simulink model "LQR_Simulink_Model"  (R2021a)
settings: Solver=VariableStepAuto  StartTime=0.0  StopTime=30  RelTol=1e-3
values from neighbouring files (symbols this model uses):
  f = 0.01    [modeling.m]
  g = 9.81    [modeling.m]
  I_pend = 0.00024    [modeling.m]
  K = K/v_to_force    [modeling.m]
  l = 0.04    [modeling.m]
  m_cart = 0.493    [modeling.m]
  m_pend = 0.312    [modeling.m]
libraries: simulink x1
settings Model: Creator=navoditchandra  LastModifiedBy=INEEDHEALING
settings DebuggingCC: UnderSpecifiedDimensionMsg=warning

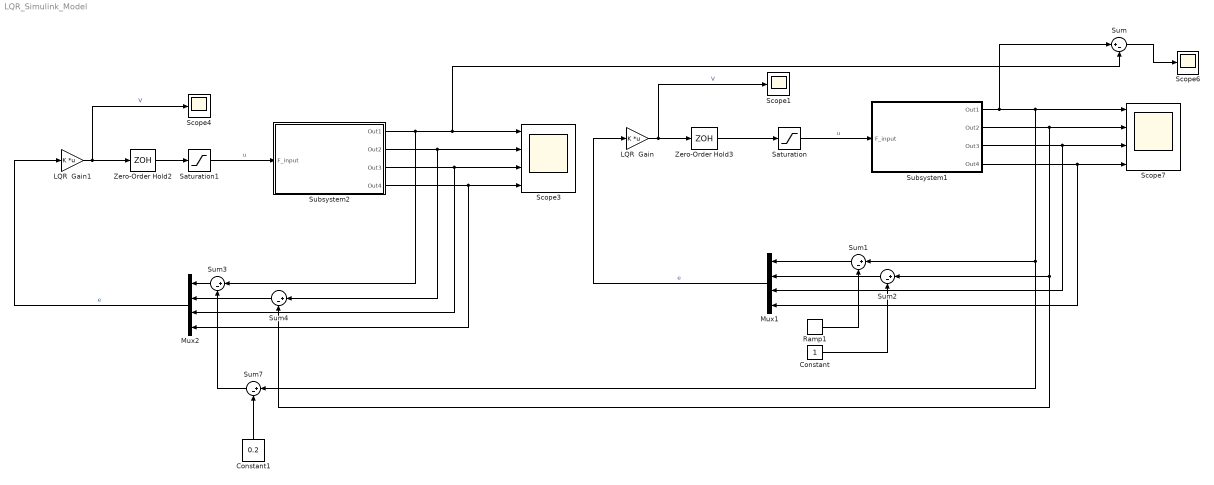
== system LQR_Simulink_Model ==
  Constant : Constant
  Constant1 : Constant  Value=0.2
  LQR  Gain : Gain  Gain=K  Multiplication=Matrix(K*u)
  LQR  Gain1 : Gain  Gain=K  Multiplication=Matrix(K*u)
  Mux1 : Mux
  Mux2 : Mux
  Ramp1 : simulink/Sources/Ramp  slope=1  start=0  InitialOutput=0
  Saturation : Saturate  UpperLimit=5  LowerLimit=-5
  Saturation1 : Saturate  UpperLimit=5  LowerLimit=-5
  Scope1 : Scope
  Scope3 : Scope  NumInputPorts=4
  Scope4 : Scope
  Scope6 : Scope
  Scope7 : Scope  NumInputPorts=4
  Subsystem1 : Subsystem
  Subsystem2 : Subsystem
  Sum{,1..4,7} (6 alike) : Sum  Inputs=|+-
  Zero-Order Hold2 : ZeroOrderHold  SampleTime=0.01
  Zero-Order Hold3 : ZeroOrderHold  SampleTime=0.01
  wires:
  Sum4/1 -> Mux2/2
  Sum3/1 -> Mux2/1
  Subsystem1/2(Out2) -> Scope7/2, Sum2/1, Sum4/2
  Mux1/1 -> LQR  Gain/1  "e"
  Subsystem1/4(Out4) -> Scope7/4, Mux1/4
  Saturation1/1 -> Subsystem2/1(F_input)  "u"
  Ramp1/1 -> Sum1/2
  Subsystem2/4(Out4) -> Mux2/4, Scope3/4
  Subsystem2/3(Out3) -> Mux2/3, Scope3/3
  Sum2/1 -> Mux1/2
  Mux2/1 -> LQR  Gain1/1  "e"
  Subsystem1/3(Out3) -> Scope7/3, Mux1/3
  Subsystem2/1(Out1) -> Scope3/1, Sum/2, Sum3/1
  Sum/1 -> Scope6/1
  Sum1/1 -> Mux1/1
  Subsystem2/2(Out2) -> Sum4/1, Scope3/2
  Subsystem1/1(Out1) -> Scope7/1, Sum7/1, Sum1/1, Sum/1
  Saturation/1 -> Subsystem1/1(F_input)  "u"
  Constant/1 -> Sum2/2
  Sum7/1 -> Sum3/2
  Constant1/1 -> Sum7/2
  LQR  Gain1/1 -> Scope4/1, Zero-Order Hold2/1  "V"
  Zero-Order Hold2/1 -> Saturation1/1
  LQR  Gain/1 -> Scope1/1, Zero-Order Hold3/1  "V"
  Zero-Order Hold3/1 -> Saturation/1

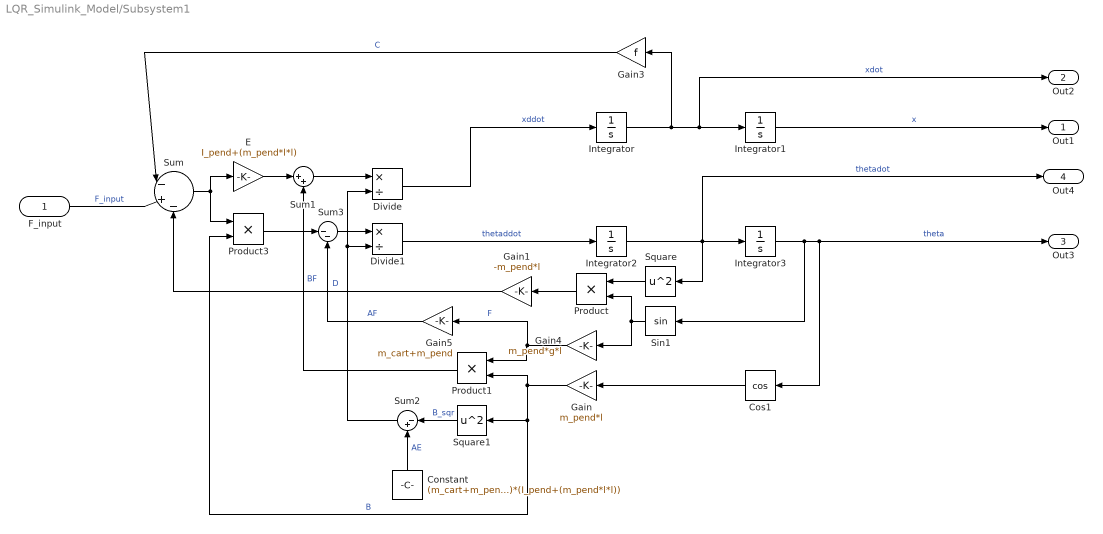
== system LQR_Simulink_Model/Subsystem1 ==
  F_input : Inport
  Constant : Constant  Value=(m_cart+m_pend)*(I_pend+(m_pend*l*l))
  Cos1 : Trigonometry  Operator=cos
  Divide : Product  Inputs=*/
  Divide1 : Product  Inputs=*/
  E : Gain  Gain=I_pend+(m_pend*l*l)
  Gain : Gain  Gain=m_pend*l
  Gain1 : Gain  Gain=-m_pend*l
  Gain3 : Gain  Gain=f
  Gain4 : Gain  Gain=m_pend*g*l
  Gain5 : Gain  Gain=m_cart+m_pend
  Integrator{,1..3} (4 alike) : Integrator
  Product : Product
  Product1 : Product
  Product3 : Product
  Sin1 : Trigonometry
  Square : Math  Operator=square  SaturateOnIntegerOverflow=on
  Square1 : Math  Operator=square  SaturateOnIntegerOverflow=on
  Sum : Sum  Inputs=|-+-
  Sum1 : Sum  Inputs=|++
  Sum2 : Sum  Inputs=|-+
  Sum3 : Sum  Inputs=|--
  Out1 : Outport
  Out2 : Outport  Port=2
  Out3 : Outport  Port=3
  Out4 : Outport  Port=4
  wires:
  Integrator2/1 -> Out4/1, Integrator3/1, Square/1  "thetadot"
  Integrator/1 -> Gain3/1, Integrator1/1, Out2/1  "xdot"
  Divide/1 -> Integrator/1  "xddot"
  Divide1/1 -> Integrator2/1  "thetaddot"
  Integrator1/1 -> Out1/1  "x"
  Gain/1 -> Product1/2, Product3/2, Square1/1  "B"
  Cos1/1 -> Gain/1
  Integrator3/1 -> Out3/1, Cos1/1, Sin1/1  "theta"
  Gain3/1 -> Sum/1  "C"
  Sin1/1 -> Gain4/1, Product/2
  Square/1 -> Product/1
  Product/1 -> Gain1/1
  Gain1/1 -> Sum/3  "D"
  Gain4/1 -> Gain5/1, Product1/1  "F"
  F_input/1 -> Sum/2  "F_input"
  Sum/1 -> Product3/1, E/1
  E/1 -> Sum1/1
  Product1/1 -> Sum1/2  "BF"
  Sum1/1 -> Divide/1
  Square1/1 -> Sum2/1  "B_sqr"
  Constant/1 -> Sum2/2  "AE"
  Sum2/1 -> Divide/2, Divide1/2
  Product3/1 -> Sum3/1
  Gain5/1 -> Sum3/2  "AF"
  Sum3/1 -> Divide1/1

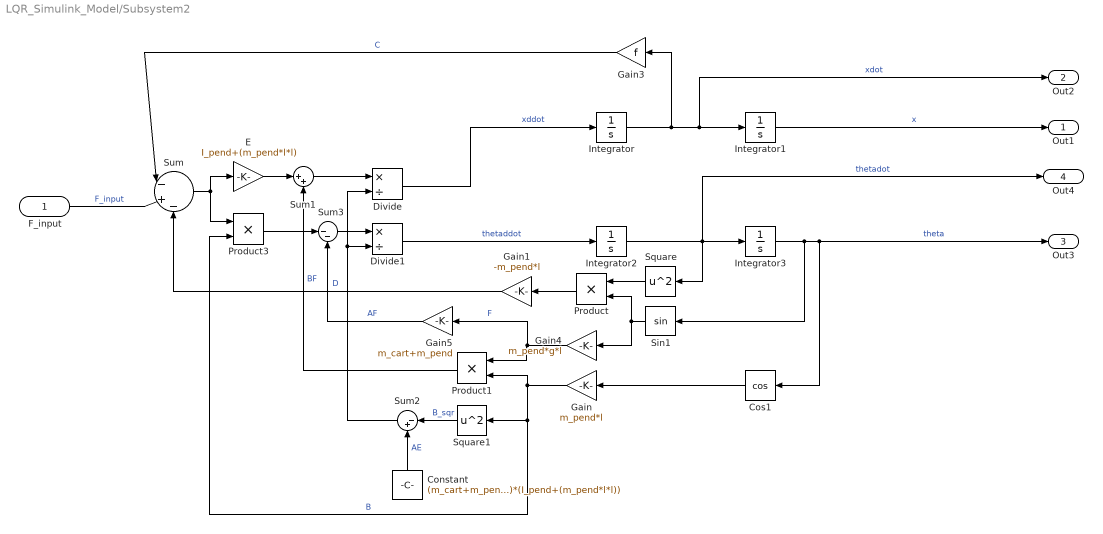
== system LQR_Simulink_Model/Subsystem2 ==
  F_input : Inport
  Constant : Constant  Value=(m_cart+m_pend)*(I_pend+(m_pend*l*l))
  Cos1 : Trigonometry  Operator=cos
  Divide : Product  Inputs=*/
  Divide1 : Product  Inputs=*/
  E : Gain  Gain=I_pend+(m_pend*l*l)
  Gain : Gain  Gain=m_pend*l
  Gain1 : Gain  Gain=-m_pend*l
  Gain3 : Gain  Gain=f
  Gain4 : Gain  Gain=m_pend*g*l
  Gain5 : Gain  Gain=m_cart+m_pend
  Integrator : Integrator
  Integrator1 : Integrator  InitialCondition=-0.2
  Integrator2 : Integrator
  Integrator3 : Integrator
  Product : Product
  Product1 : Product
  Product3 : Product
  Sin1 : Trigonometry
  Square : Math  Operator=square  SaturateOnIntegerOverflow=on
  Square1 : Math  Operator=square  SaturateOnIntegerOverflow=on
  Sum : Sum  Inputs=|-+-
  Sum1 : Sum  Inputs=|++
  Sum2 : Sum  Inputs=|-+
  Sum3 : Sum  Inputs=|--
  Out1 : Outport
  Out2 : Outport  Port=2
  Out3 : Outport  Port=3
  Out4 : Outport  Port=4
  wires:
  Integrator2/1 -> Out4/1, Integrator3/1, Square/1  "thetadot"
  Integrator/1 -> Gain3/1, Integrator1/1, Out2/1  "xdot"
  Divide/1 -> Integrator/1  "xddot"
  Divide1/1 -> Integrator2/1  "thetaddot"
  Integrator1/1 -> Out1/1  "x"
  Gain/1 -> Product1/2, Product3/2, Square1/1  "B"
  Cos1/1 -> Gain/1
  Integrator3/1 -> Out3/1, Cos1/1, Sin1/1  "theta"
  Gain3/1 -> Sum/1  "C"
  Sin1/1 -> Gain4/1, Product/2
  Square/1 -> Product/1
  Product/1 -> Gain1/1
  Gain1/1 -> Sum/3  "D"
  Gain4/1 -> Gain5/1, Product1/1  "F"
  F_input/1 -> Sum/2  "F_input"
  Sum/1 -> Product3/1, E/1
  E/1 -> Sum1/1
  Product1/1 -> Sum1/2  "BF"
  Sum1/1 -> Divide/1
  Square1/1 -> Sum2/1  "B_sqr"
  Constant/1 -> Sum2/2  "AE"
  Sum2/1 -> Divide/2, Divide1/2
  Product3/1 -> Sum3/1
  Gain5/1 -> Sum3/2  "AF"
  Sum3/1 -> Divide1/1
